simulink model "simulink_deadbeat_control101_2024"  (R2024a)
settings: Solver=VariableStepAuto  StartTime=0.0  StopTime=endtime  RelTol=1e-3
undefined symbols (not defined in the file or in its folder): deadtime, tplot, Ts
libraries: cstblocks x2
settings Model: Creator=barsr  LastModifiedBy=Anthony Rossiter
settings RTWCC: GPUComputeCapability=3.5

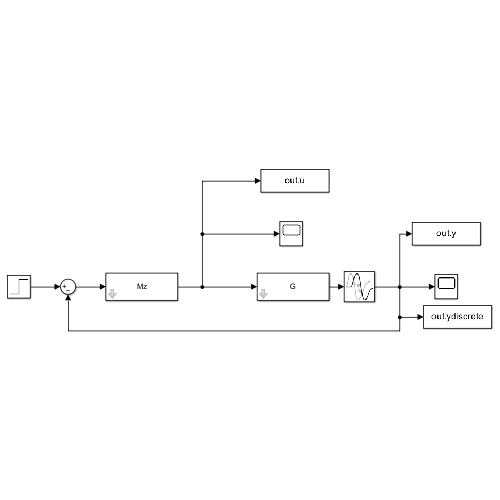
[thumbnail: Simulink's stored preview of the top-level diagram]
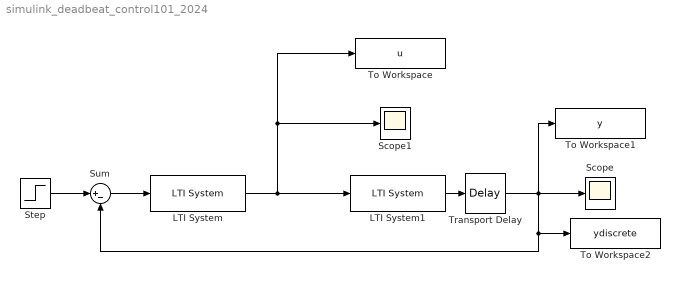
== system simulink_deadbeat_control101_2024 ==
  LTI System : cstblocks/LTI System  sys=Mz  IC=[]  PadeOrder=0
  LTI System1 : cstblocks/LTI System  sys=G  IC=[]  PadeOrder=0
  Scope : Scope
  Scope1 : Scope
  Step : Step  Time=0  SampleTime=0
  Sum : Sum  Inputs=|+-
  To Workspace : ToWorkspace  VariableName=u  SaveFormat=Structure With Time  SampleTime=tplot
  To Workspace1 : ToWorkspace  VariableName=y  SaveFormat=Structure With Time  SampleTime=tplot
  To Workspace2 : ToWorkspace  VariableName=ydiscrete  SaveFormat=Structure With Time  SampleTime=Ts
  Transport Delay : TransportDelay  DelayTime=deadtime
  wires:
  Step/1 -> Sum/1
  Sum/1 -> LTI System/1
  Transport Delay/1 -> To Workspace1/1, Sum/2, To Workspace2/1, Scope/1
  LTI System1/1 -> Transport Delay/1
  LTI System/1 -> To Workspace/1, Scope1/1, LTI System1/1
